simulink model "ControladorRetroDiscreto(1)"  (R2022b)
settings: Solver=VariableStepAuto  StartTime=0.0  StopTime=10  RelTol=1e-3
values from neighbouring files (symbols this model uses):
  C = tf(Kc*[ti*td ti 1],[ti 0])    [PID_Ku.m]    (also in Raices.m = (s^2+2*zeta*wn*s+wn^2)/(0.1*s+1); Routh_Hurwitz.m = [1 0 0]; Smulacro_Parcial_Final.m = matrizC; diseñoCompensadorAdelanto.m = leadlag(K, Td, Ti))
undefined symbols (not defined in the file or in its folder): Gev, H1, k13ev, ke, kiev
settings Model: Creator=Juan  LastModifiedBy=Duván Ramírez Lotta
settings ModelReferenceCC: EnableRefExpFcnMdlSchedulingChecks=on

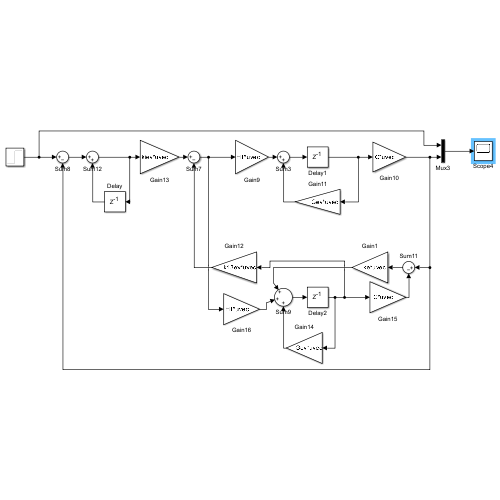
[thumbnail: Simulink's stored preview of the top-level diagram]
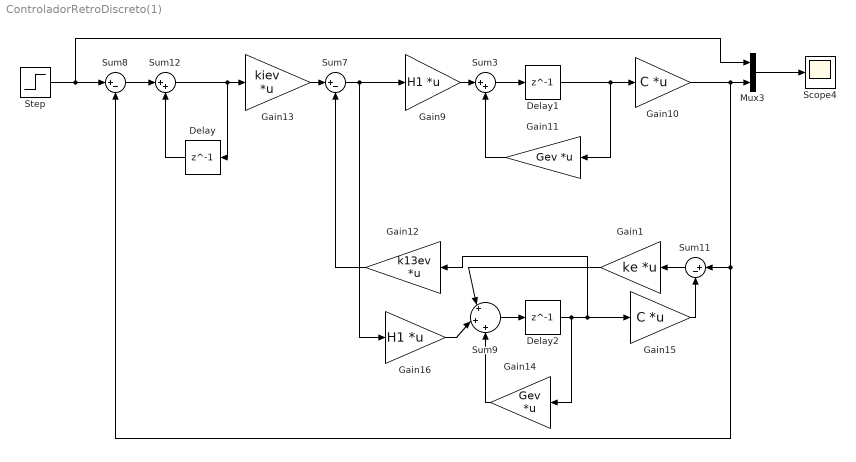
== system ControladorRetroDiscreto(1) ==
  Delay : Delay  DelayLength=1  SampleTime=0.001
  Delay1 : Delay  DelayLength=1  SampleTime=0.001
  Delay2 : Delay  DelayLength=1  SampleTime=0.001
  Gain1 : Gain  Gain=ke  Multiplication=Matrix(K*u) (u vector)
  Gain10 : Gain  Gain=C  Multiplication=Matrix(K*u) (u vector)
  Gain11 : Gain  Gain=Gev  Multiplication=Matrix(K*u) (u vector)
  Gain12 : Gain  Gain=k13ev  Multiplication=Matrix(K*u) (u vector)
  Gain13 : Gain  Gain=kiev  Multiplication=Matrix(K*u) (u vector)
  Gain14 : Gain  Gain=Gev  Multiplication=Matrix(K*u) (u vector)
  Gain15 : Gain  Gain=C  Multiplication=Matrix(K*u) (u vector)
  Gain16 : Gain  Gain=H1  Multiplication=Matrix(K*u) (u vector)
  Gain9 : Gain  Gain=H1  Multiplication=Matrix(K*u) (u vector)
  Mux3 : Mux  Inputs=2
  Scope4 : Scope
  Step : Step  SampleTime=0
  Sum11 : Sum  Inputs=|+-
  Sum12 : Sum  Inputs=|++
  Sum3 : Sum  Inputs=|++
  Sum7 : Sum  Inputs=|+-
  Sum8 : Sum  Inputs=|+-
  Sum9 : Sum  Inputs=|+|+|+
  wires:
  Sum3/1 -> Delay1/1
  Sum8/1 -> Sum12/1
  Sum7/1 -> Gain16/1, Gain9/1
  Gain9/1 -> Sum3/1
  Mux3/1 -> Scope4/1
  Step/1 -> Mux3/1, Sum8/1
  Gain11/1 -> Sum3/2
  Gain10/1 -> Mux3/2, Sum11/1, Sum8/2
  Gain13/1 -> Sum7/1
  Sum12/1 -> Delay/1, Gain13/1
  Delay/1 -> Sum12/2
  Delay1/1 -> Gain11/1, Gain10/1
  Gain12/1 -> Sum7/2
  Gain15/1 -> Sum11/2
  Delay2/1 -> Gain14/1, Gain12/1, Gain15/1
  Sum9/1 -> Delay2/1
  Gain14/1 -> Sum9/3
  Gain16/1 -> Sum9/2
  Sum11/1 -> Gain1/1
  Gain1/1 -> Sum9/1
